simulink model "SimModeleNonLineaire"  (R2018b)
settings: Solver=VariableStepAuto  StartTime=0.0  StopTime=10.0  RelTol=1e-3
undefined symbols (not defined in the file): ae0, ae1, ae2, ae3, as0, as1, as2, as3, be1, g, JS, Jx, Jy, L, mS, mSg, mtot, R, rS, Vmax, XA, XB, XC, YA, YB, YC
settings Model: Creator=Vincent  LastModifiedBy=Vincent

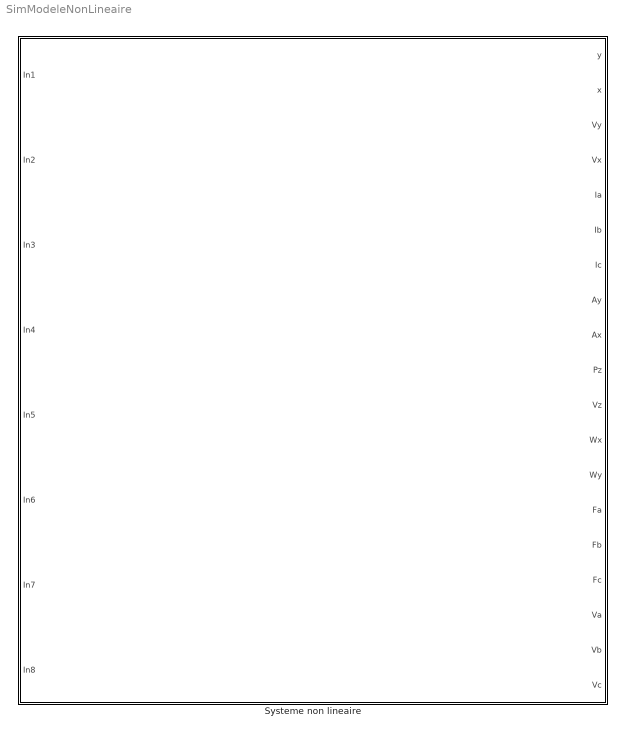
== system SimModeleNonLineaire ==
  Systeme non lineaire : Subsystem

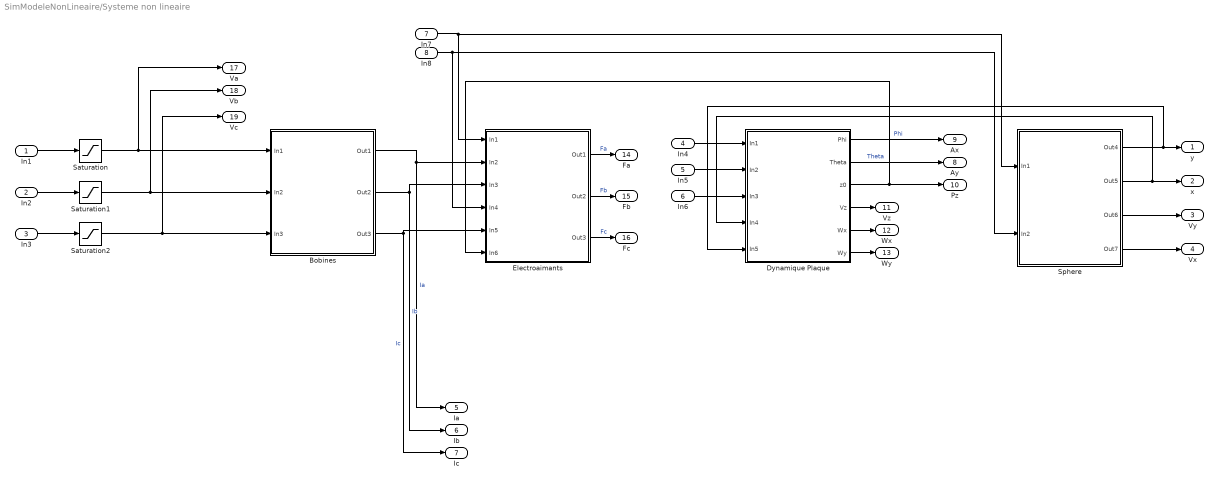
== system SimModeleNonLineaire/Systeme non lineaire ==
  In1 : Inport
  In2 : Inport  Port=2
  In3 : Inport  Port=3
  In4 : Inport  Port=4
  In5 : Inport  Port=5
  In6 : Inport  Port=6
  In7 : Inport  Port=7
  In8 : Inport  Port=8
  Bobines : Subsystem
  Dynamique Plaque : Subsystem
  Electroaimants : Subsystem
  Saturation : Saturate  UpperLimit=Vmax  LowerLimit=-Vmax
  Saturation1 : Saturate  UpperLimit=Vmax  LowerLimit=-Vmax
  Saturation2 : Saturate  UpperLimit=Vmax  LowerLimit=-Vmax
  Sphere : Subsystem
  y : Outport
  x : Outport  Port=2
  Vy : Outport  Port=3
  Vx : Outport  Port=4
  Ia : Outport  Port=5
  Ib : Outport  Port=6
  Ic : Outport  Port=7
  Ay : Outport  Port=8
  Ax : Outport  Port=9
  Pz : Outport  Port=10
  Vz : Outport  Port=11
  Wx : Outport  Port=12
  Wy : Outport  Port=13
  Fa : Outport  Port=14
  Fb : Outport  Port=15
  Fc : Outport  Port=16
  Va : Outport  Port=17
  Vb : Outport  Port=18
  Vc : Outport  Port=19
  wires:
  Electroaimants/2(Out2) -> Fb/1  "Fb"
  Bobines/2(Out2) -> Ib/1, Electroaimants/3(In3)  "Ib"
  Bobines/1(Out1) -> Electroaimants/2(In2), Ia/1  "Ia"
  Dynamique Plaque/2(Theta) -> Ay/1  "Theta"
  In2/1 -> Saturation1/1
  Electroaimants/1(Out1) -> Fa/1  "Fa"
  In1/1 -> Saturation/1
  Electroaimants/3(Out3) -> Fc/1  "Fc"
  Dynamique Plaque/1(Phi) -> Ax/1  "Phi"
  Bobines/3(Out3) -> Ic/1, Electroaimants/5(In5)  "Ic"
  In3/1 -> Saturation2/1
  Sphere/1(Out4) -> y/1, Dynamique Plaque/5(In5)
  Sphere/2(Out5) -> Dynamique Plaque/4(In4), x/1
  Sphere/3(Out6) -> Vy/1
  Sphere/4(Out7) -> Vx/1
  Dynamique Plaque/4(Vz) -> Vz/1
  Dynamique Plaque/5(Wx) -> Wx/1
  Dynamique Plaque/6(Wy) -> Wy/1
  Saturation/1 -> Bobines/1(In1), Va/1
  Saturation2/1 -> Bobines/3(In3), Vc/1
  Saturation1/1 -> Bobines/2(In2), Vb/1
  Dynamique Plaque/3(z0) -> Pz/1, Electroaimants/6(In6)
  In4/1 -> Dynamique Plaque/1(In1)
  In5/1 -> Dynamique Plaque/2(In2)
  In6/1 -> Dynamique Plaque/3(In3)
  In8/1 -> Electroaimants/4(In4), Sphere/2(In2)
  In7/1 -> Sphere/1(In1), Electroaimants/1(In1)

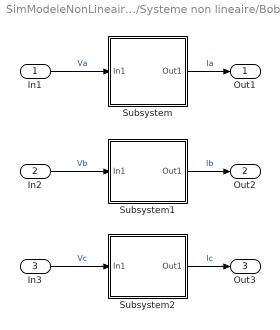
== system SimModeleNonLineaire/Systeme non lineaire/Bobines ==
  In1 : Inport
  In2 : Inport  Port=2
  In3 : Inport  Port=3
  Subsystem : Subsystem
  Subsystem1 : Subsystem
  Subsystem2 : Subsystem
  Out1 : Outport
  Out2 : Outport  Port=2
  Out3 : Outport  Port=3
  wires:
  In1/1 -> Subsystem/1(In1)  "Va"
  In2/1 -> Subsystem1/1(In1)  "Vb"
  Subsystem2/1(Out1) -> Out3/1  "Ic"
  Subsystem/1(Out1) -> Out1/1  "Ia"
  In3/1 -> Subsystem2/1(In1)  "Vc"
  Subsystem1/1(Out1) -> Out2/1  "Ib"

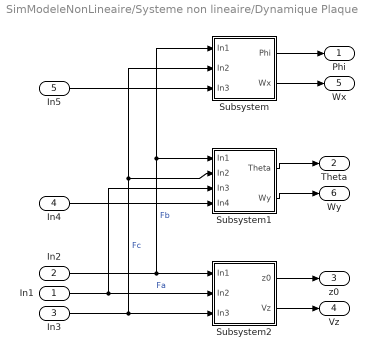
== system SimModeleNonLineaire/Systeme non lineaire/Dynamique Plaque ==
  In1 : Inport
  In2 : Inport  Port=2
  In3 : Inport  Port=3
  In4 : Inport  Port=4
  In5 : Inport  Port=5
  Subsystem : Subsystem
  Subsystem1 : Subsystem
  Subsystem2 : Subsystem
  Phi : Outport
  Theta : Outport  Port=2
  z0 : Outport  Port=3
  Vz : Outport  Port=4
  Wx : Outport  Port=5
  Wy : Outport  Port=6
  wires:
  In1/1 -> Subsystem1/3(In3), Subsystem2/2(In2)  "Fa"
  In3/1 -> Subsystem/2(In2), Subsystem1/2(In2), Subsystem2/3(In3)  "Fc"
  Subsystem1/1(Theta) -> Theta/1
  In2/1 -> Subsystem1/1(In1), Subsystem/1(In1), Subsystem2/1(In1)  "Fb"
  Subsystem/1(Phi) -> Phi/1
  Subsystem2/1(z0) -> z0/1
  Subsystem2/2(Vz) -> Vz/1
  Subsystem/2(Wx) -> Wx/1
  Subsystem1/2(Wy) -> Wy/1
  In4/1 -> Subsystem1/4(In4)
  In5/1 -> Subsystem/3(In3)

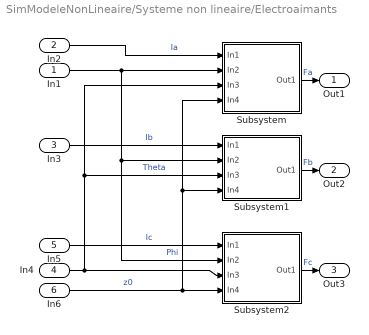
== system SimModeleNonLineaire/Systeme non lineaire/Electroaimants ==
  In1 : Inport
  In2 : Inport  Port=2
  In3 : Inport  Port=3
  In4 : Inport  Port=4
  In5 : Inport  Port=5
  In6 : Inport  Port=6
  Subsystem : Subsystem
  Subsystem1 : Subsystem
  Subsystem2 : Subsystem
  Out1 : Outport
  Out2 : Outport  Port=2
  Out3 : Outport  Port=3
  wires:
  In6/1 -> Subsystem2/4(In4), Subsystem1/4(In4), Subsystem/4(In4)  "z0"
  In4/1 -> Subsystem2/3(In3), Subsystem/3(In3), Subsystem1/3(In3)  "Theta"
  In5/1 -> Subsystem2/1(In1)  "Ic"
  In1/1 -> Subsystem/2(In2), Subsystem2/2(In2), Subsystem1/2(In2)  "Phi"
  Subsystem2/1(Out1) -> Out3/1  "Fc"
  In2/1 -> Subsystem/1(In1)  "Ia"
  In3/1 -> Subsystem1/1(In1)  "Ib"
  Subsystem1/1(Out1) -> Out2/1  "Fb"
  Subsystem/1(Out1) -> Out1/1  "Fa"

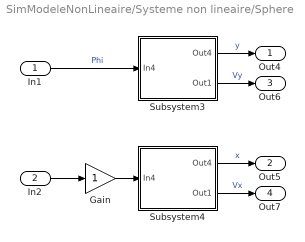
== system SimModeleNonLineaire/Systeme non lineaire/Sphere ==
  In1 : Inport
  In2 : Inport  Port=2
  Gain : Gain
  Subsystem3 : Subsystem
  Subsystem4 : Subsystem
  Out4 : Outport
  Out5 : Outport  Port=2
  Out6 : Outport  Port=3
  Out7 : Outport  Port=4
  wires:
  Subsystem3/2(Out1) -> Out6/1  "Vy"
  Subsystem4/1(Out4) -> Out5/1  "x"
  Subsystem3/1(Out4) -> Out4/1  "y"
  In2/1 -> Gain/1
  Subsystem4/2(Out1) -> Out7/1  "Vx"
  Gain/1 -> Subsystem4/1(In4)
  In1/1 -> Subsystem3/1(In4)  "Phi"

== system SimModeleNonLineaire/Systeme non lineaire/Bobines/Subsystem ==
  note: Ia
  note: Va
  In1 : Inport
  Gain : Gain  Gain=1/L
  Gain1 : Gain  Gain=R/L
  Integrator : Integrator
  Sum : Sum  Inputs=|+-
  Out1 : Outport
  wires:
  Integrator/1 -> Out1/1, Gain1/1
  Gain/1 -> Sum/1
  Gain1/1 -> Sum/2
  Sum/1 -> Integrator/1
  In1/1 -> Gain/1

== system SimModeleNonLineaire/Systeme non lineaire/Bobines/Subsystem1 ==
  In1 : Inport
  Gain : Gain  Gain=1/L
  Gain1 : Gain  Gain=R/L
  Integrator : Integrator
  Sum : Sum  Inputs=|+-
  Out1 : Outport
  wires:
  Integrator/1 -> Out1/1, Gain1/1
  Gain/1 -> Sum/1
  Gain1/1 -> Sum/2
  Sum/1 -> Integrator/1
  In1/1 -> Gain/1

== system SimModeleNonLineaire/Systeme non lineaire/Bobines/Subsystem2 ==
  In1 : Inport
  Gain : Gain  Gain=1/L
  Gain1 : Gain  Gain=R/L
  Integrator : Integrator
  Sum : Sum  Inputs=|+-
  Out1 : Outport
  wires:
  Integrator/1 -> Out1/1, Gain1/1
  Gain/1 -> Sum/1
  Gain1/1 -> Sum/2
  Sum/1 -> Integrator/1
  In1/1 -> Gain/1

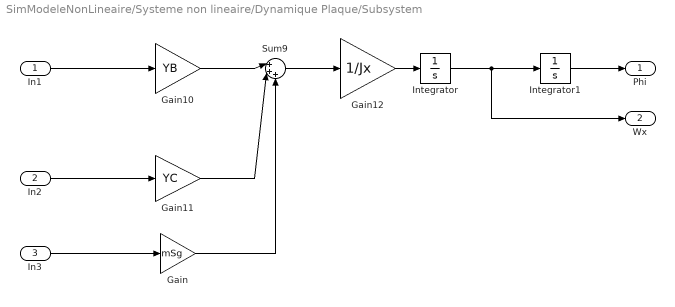
== system SimModeleNonLineaire/Systeme non lineaire/Dynamique Plaque/Subsystem ==
  In1 : Inport
  In2 : Inport  Port=2
  In3 : Inport  Port=3
  Gain : Gain  Gain=mSg
  Gain10 : Gain  Gain=YB
  Gain11 : Gain  Gain=YC
  Gain12 : Gain  Gain=1/Jx
  Integrator : Integrator
  Integrator1 : Integrator
  Sum9 : Sum  Inputs=|+++
  Phi : Outport
  Wx : Outport  Port=2
  wires:
  Integrator1/1 -> Phi/1
  In2/1 -> Gain11/1
  Integrator/1 -> Wx/1, Integrator1/1
  Gain10/1 -> Sum9/1
  Sum9/1 -> Gain12/1
  Gain12/1 -> Integrator/1
  Gain11/1 -> Sum9/2
  In1/1 -> Gain10/1
  Gain/1 -> Sum9/3
  In3/1 -> Gain/1

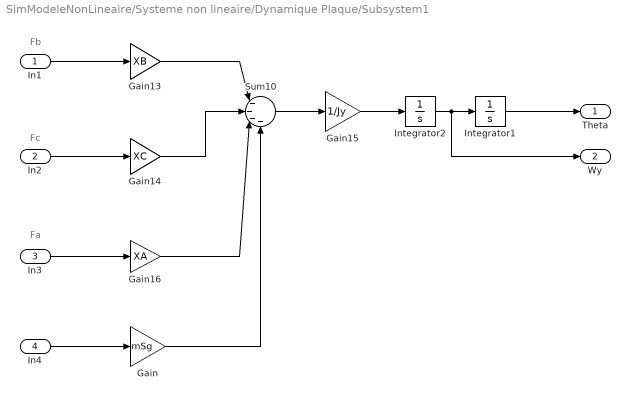
== system SimModeleNonLineaire/Systeme non lineaire/Dynamique Plaque/Subsystem1 ==
  note: Fa
  note: Fc
  note: Fb
  In1 : Inport
  In2 : Inport  Port=2
  In3 : Inport  Port=3
  In4 : Inport  Port=4
  Gain : Gain  Gain=mSg
  Gain13 : Gain  Gain=XB
  Gain14 : Gain  Gain=XC
  Gain15 : Gain  Gain=1/Jy
  Gain16 : Gain  Gain=XA
  Integrator1 : Integrator
  Integrator2 : Integrator
  Sum10 : Sum  Inputs=|----
  Theta : Outport
  Wy : Outport  Port=2
  wires:
  In3/1 -> Gain16/1
  Gain14/1 -> Sum10/2
  Gain15/1 -> Integrator2/1
  Sum10/1 -> Gain15/1
  In1/1 -> Gain13/1
  Gain13/1 -> Sum10/1
  Integrator2/1 -> Wy/1, Integrator1/1
  In2/1 -> Gain14/1
  Gain16/1 -> Sum10/3
  Integrator1/1 -> Theta/1
  In4/1 -> Gain/1
  Gain/1 -> Sum10/4

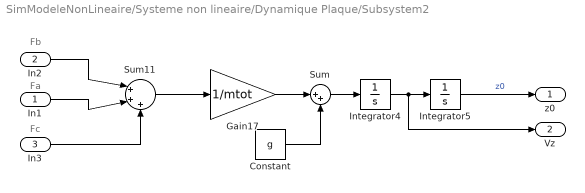
== system SimModeleNonLineaire/Systeme non lineaire/Dynamique Plaque/Subsystem2 ==
  note: Fc
  note: Fa
  note: Fb
  In1 : Inport
  In2 : Inport  Port=2
  In3 : Inport  Port=3
  Constant : Constant  Value=g
  Gain17 : Gain  Gain=1/mtot
  Integrator4 : Integrator
  Integrator5 : Integrator  InitialCondition=0.015
  Sum : Sum  Inputs=|++
  Sum11 : Sum  Inputs=|+++
  z0 : Outport
  Vz : Outport  Port=2
  wires:
  Integrator5/1 -> z0/1  "z0"
  In3/1 -> Sum11/3
  Sum11/1 -> Gain17/1
  In1/1 -> Sum11/2
  Integrator4/1 -> Vz/1, Integrator5/1
  Gain17/1 -> Sum/1
  In2/1 -> Sum11/1
  Sum/1 -> Integrator4/1
  Constant/1 -> Sum/2

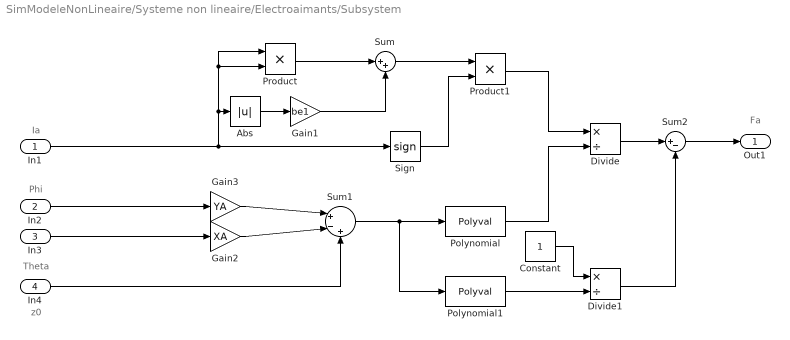
== system SimModeleNonLineaire/Systeme non lineaire/Electroaimants/Subsystem ==
  note: Fa
  note: z0
  note: Theta
  note: Phi
  note: Ia
  In1 : Inport
  In2 : Inport  Port=2
  In3 : Inport  Port=3
  In4 : Inport  Port=4
  Abs : Abs
  Constant : Constant
  Divide : Product  Inputs=*/
  Divide1 : Product  Inputs=*/
  Gain1 : Gain  Gain=be1
  Gain2 : Gain  Gain=XA
  Gain3 : Gain  Gain=YA
  Polynomial : Polyval  Coefs=[ae3 ae2 ae1 ae0]
  Polynomial1 : Polyval  Coefs=[as3 as2 as1 as0]
  Product : Product
  Product1 : Product
  Sign : Signum
  Sum : Sum  Inputs=|++
  Sum1 : Sum  Inputs=|+-+
  Sum2 : Sum  Inputs=|+-
  Out1 : Outport
  wires:
  Sum/1 -> Product1/1
  Product1/1 -> Divide/1
  Gain2/1 -> Sum1/2
  Sum2/1 -> Out1/1
  Constant/1 -> Divide1/1
  Product/1 -> Sum/1
  Polynomial/1 -> Divide/2
  In1/1 -> Product/1, Product/2, Abs/1, Sign/1
  Abs/1 -> Gain1/1
  Gain1/1 -> Sum/2
  Polynomial1/1 -> Divide1/2
  Sum1/1 -> Polynomial1/1, Polynomial/1
  Sign/1 -> Product1/2
  In4/1 -> Sum1/3
  Divide/1 -> Sum2/1
  Gain3/1 -> Sum1/1
  Divide1/1 -> Sum2/2
  In2/1 -> Gain3/1
  In3/1 -> Gain2/1

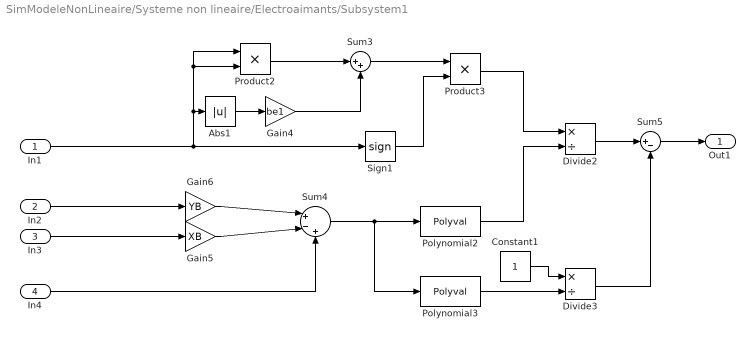
== system SimModeleNonLineaire/Systeme non lineaire/Electroaimants/Subsystem1 ==
  In1 : Inport
  In2 : Inport  Port=2
  In3 : Inport  Port=3
  In4 : Inport  Port=4
  Abs1 : Abs
  Constant1 : Constant
  Divide2 : Product  Inputs=*/
  Divide3 : Product  Inputs=*/
  Gain4 : Gain  Gain=be1
  Gain5 : Gain  Gain=XB
  Gain6 : Gain  Gain=YB
  Polynomial2 : Polyval  Coefs=[ae3 ae2 ae1 ae0]
  Polynomial3 : Polyval  Coefs=[as3 as2 as1 as0]
  Product2 : Product
  Product3 : Product
  Sign1 : Signum
  Sum3 : Sum  Inputs=|++
  Sum4 : Sum  Inputs=|+-+
  Sum5 : Sum  Inputs=|+-
  Out1 : Outport
  wires:
  In2/1 -> Gain6/1
  Gain6/1 -> Sum4/1
  In4/1 -> Sum4/3
  Gain5/1 -> Sum4/2
  Sum4/1 -> Polynomial3/1, Polynomial2/1
  In1/1 -> Product2/1, Product2/2, Abs1/1, Sign1/1
  Constant1/1 -> Divide3/1
  Sign1/1 -> Product3/2
  Divide2/1 -> Sum5/1
  In3/1 -> Gain5/1
  Divide3/1 -> Sum5/2
  Polynomial3/1 -> Divide3/2
  Product3/1 -> Divide2/1
  Gain4/1 -> Sum3/2
  Abs1/1 -> Gain4/1
  Product2/1 -> Sum3/1
  Sum3/1 -> Product3/1
  Polynomial2/1 -> Divide2/2
  Sum5/1 -> Out1/1

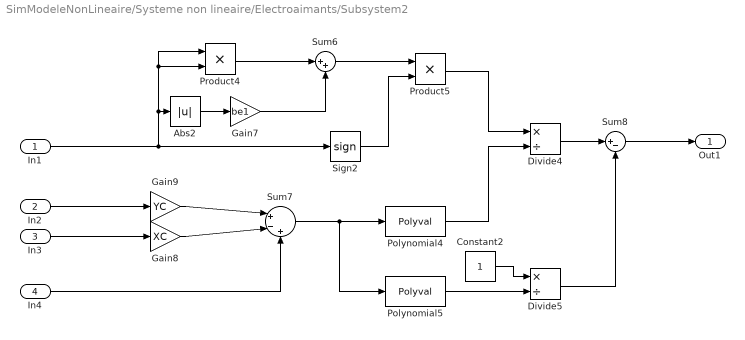
== system SimModeleNonLineaire/Systeme non lineaire/Electroaimants/Subsystem2 ==
  In1 : Inport
  In2 : Inport  Port=2
  In3 : Inport  Port=3
  In4 : Inport  Port=4
  Abs2 : Abs
  Constant2 : Constant
  Divide4 : Product  Inputs=*/
  Divide5 : Product  Inputs=*/
  Gain7 : Gain  Gain=be1
  Gain8 : Gain  Gain=XC
  Gain9 : Gain  Gain=YC
  Polynomial4 : Polyval  Coefs=[ae3 ae2 ae1 ae0]
  Polynomial5 : Polyval  Coefs=[as3 as2 as1 as0]
  Product4 : Product
  Product5 : Product
  Sign2 : Signum
  Sum6 : Sum  Inputs=|++
  Sum7 : Sum  Inputs=|+-+
  Sum8 : Sum  Inputs=|+-
  Out1 : Outport
  wires:
  Gain9/1 -> Sum7/1
  Gain8/1 -> Sum7/2
  Divide5/1 -> Sum8/2
  Divide4/1 -> Sum8/1
  Constant2/1 -> Divide5/1
  In1/1 -> Product4/1, Product4/2, Abs2/1, Sign2/1
  Sum7/1 -> Polynomial5/1, Polynomial4/1
  Sign2/1 -> Product5/2
  In2/1 -> Gain9/1
  Product4/1 -> Sum6/1
  Product5/1 -> Divide4/1
  In4/1 -> Sum7/3
  Polynomial5/1 -> Divide5/2
  Gain7/1 -> Sum6/2
  Polynomial4/1 -> Divide4/2
  Sum6/1 -> Product5/1
  Abs2/1 -> Gain7/1
  Sum8/1 -> Out1/1
  In3/1 -> Gain8/1

== system SimModeleNonLineaire/Systeme non lineaire/Sphere/Subsystem3 ==
  note: y
  note: Vy
  note: Phi
  In4 : Inport  Tag=Theta
  Gain : Gain  Gain=mS*g/(mS+JS/rS^2)
  Integrator : Integrator
  Integrator1 : Integrator
  Out4 : Outport
  Out1 : Outport  Port=2
  wires:
  Gain/1 -> Integrator/1
  In4/1 -> Gain/1
  Integrator1/1 -> Out4/1
  Integrator/1 -> Out1/1, Integrator1/1

== system SimModeleNonLineaire/Systeme non lineaire/Sphere/Subsystem4 ==
  In4 : Inport  Tag=Theta
  Gain : Gain  Gain=-mS*g/(mS+JS/rS^2)
  Integrator : Integrator
  Integrator1 : Integrator
  Out4 : Outport
  Out1 : Outport  Port=2
  wires:
  Gain/1 -> Integrator/1
  In4/1 -> Gain/1
  Integrator1/1 -> Out4/1
  Integrator/1 -> Out1/1, Integrator1/1
